simulink model "time_gongji_KVHonline_daoyuan_huace"  (R2019b)
settings: Solver=ode3  StartTime=0.0  StopTime=6000  FixedStep=0.01  MaxStep=0.01  RelTol=1e-3
values from neighbouring files (symbols this model uses):
  bias_gyro_z_gongji = 2e-3    (= 0.002)    [sych_ite_KVHonline_daoyuan_huace.m]
  g = 9.8    [sych_ite_KVHonline_daoyuan_huace.m]
settings Model: Creator=luyishi_E480  LastModifiedBy=xie_z
settings DataIOCC: SaveOutput=off  SignalLogging=off  DSMLogging=off  InspectSignalLogs=on  SaveTime=off  ReturnWorkspaceOutputs=off
settings DebuggingCC: InheritedTsInSrcMsg=none

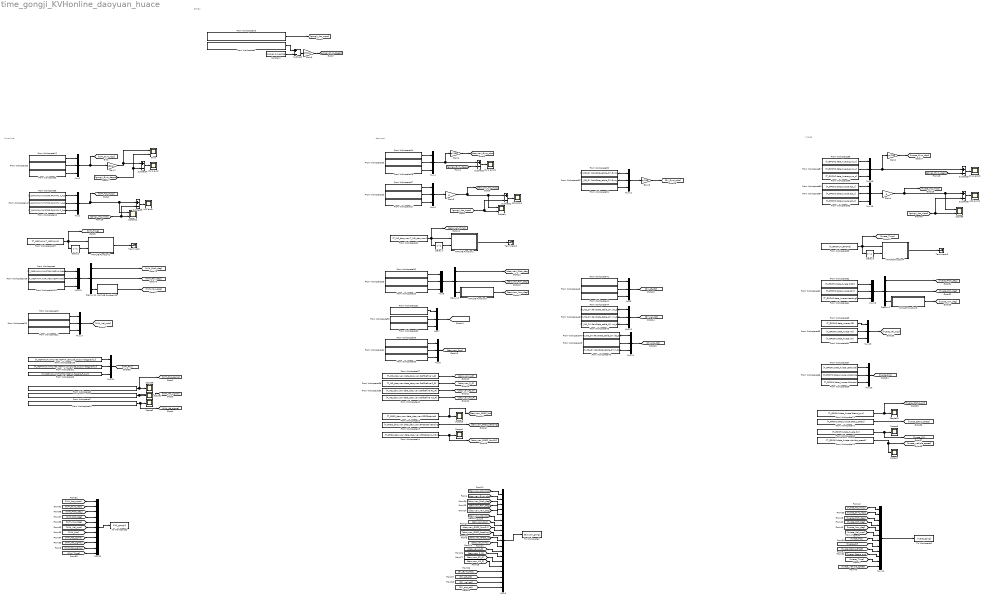
== system time_gongji_KVHonline_daoyuan_huace ==
  note: huace
  note: daoyuan
  note: gongji
  note: kvhonline
  ACC error : Scope
  ACC error1 : Scope
  ACC error2 : Scope
  Constant : Constant  Value=bias_gyro_z_gongji
  Delay1 : Delay  DelayLength=1  InitialCondition=0
  Delay2 : Delay  DelayLength=1  InitialCondition=0
  Delay3 : Delay  DelayLength=1  InitialCondition=0
  Demux1 : Demux  Outputs=3
  Demux14 : Demux  Outputs=3
  Demux2 : Demux  Outputs=3
  From Workspace1 : FromWorkspace  VariableName=[T_INSPVAXA,KVH1750.INSPVA.Longitude_Fusion*deg2rad(1)]  OutputAfterFinalValue=Holding final value
  From Workspace10 : FromWorkspace  VariableName=[T_RAWIMU,KVH1750.RAWIMU.Z_Acc]  Interpolate=off  OutputAfterFinalValue=Holding final value
  From Workspace103 : FromWorkspace  VariableName=[T_INSPVAXA,KVH1750.INSPVA.Latitude_Fusion*deg2rad(1)]  OutputAfterFinalValue=Holding final value
  From Workspace108 : FromWorkspace  VariableName=[T_INSPVAXA,KVH1750.INSPVA.Roll]  Interpolate=off  OutputAfterFinalValue=Holding final value
  From Workspace109 : FromWorkspace  VariableName=[T_INSPVAXA,T_INSPVAXA]  Interpolate=off  OutputAfterFinalValue=Holding final value
  From Workspace11 : FromWorkspace  VariableName=[T_RAWIMU,KVH1750.RAWIMU.Y_Acc]  Interpolate=off  OutputAfterFinalValue=Holding final value
  From Workspace110 : FromWorkspace  VariableName=[T_INSPVAXA,KVH1750.INSPVA.Azimuth]  Interpolate=off  OutputAfterFinalValue=Holding final value
  From Workspace12 : FromWorkspace  VariableName=[T_RAWIMU,KVH1750.RAWIMU.X_Gyro]  Interpolate=off  OutputAfterFinalValue=Holding final value
  From Workspace13 : FromWorkspace  VariableName=[T_INSPVAXA,KVH1750.INSPVA.Pitch_sigma_Fusion,KVH1750.INSPVA.Roll_sigma_Fusion,KVH1750.INSPVA.Azimuth_sigma_Fusion]  Interpolate=off  OutputAfterFinalValue=Holding final value
  From Workspace14 : FromWorkspace  VariableName=[T_GNSS_daoyuan,data_daoyuan.GPSData.NumSV]  Interpolate=off  OutputAfterFinalValue=Holding final value
  From Workspace15 : FromWorkspace  VariableName=[T_GNSS_daoyuan,data_daoyuan.GPSData.heading]  Interpolate=off  OutputAfterFinalValue=Holding final value
  From Workspace16 : FromWorkspace  VariableName=[T_GNSS_daoyuan,data_daoyuan.GPSData.Lat]  Interpolate=off  OutputAfterFinalValue=Holding final value
  From Workspace17 : FromWorkspace  VariableName=[T_INS_daoyuan,-data_daoyuan.INSData.a(:,3)]  Interpolate=off  OutputAfterFinalValue=Holding final value
  From Workspace18 : FromWorkspace  VariableName=[Time,RawData_table.IMU_ACC_x,RawData_table.IMU_ACC_y,RawData_table.IMU_ACC_z]  Interpolate=off  OutputAfterFinalValue=Holding final value
  From Workspace19 : FromWorkspace  VariableName=[T_INSPVAXA,KVH1750.INSPVA.Vel_E_Fusion]  Interpolate=off  OutputAfterFinalValue=Holding final value
  From Workspace2 : FromWorkspace  VariableName=[Time,RawData_table.IMU_Gyro_x,RawData_table.IMU_Gyro_y,RawData_table.IMU_Gyro_z]  Interpolate=off  OutputAfterFinalValue=Holding final value
  From Workspace20 : FromWorkspace  VariableName=[T_INSPVAXA,KVH1750.INSPVA.Vel_N_Fusion]  Interpolate=off  OutputAfterFinalValue=Holding final value
  From Workspace21 : FromWorkspace  VariableName=[T_INSPVAXA,KVH1750.INSPVA.Vel_U_Fusion]  Interpolate=off  OutputAfterFinalValue=Holding final value
  From Workspace22 : FromWorkspace  VariableName=[T_INS_daoyuan,T_INS_daoyuan]  Interpolate=off  OutputAfterFinalValue=Holding final value
  From Workspace23 : FromWorkspace  VariableName=[T_INS_daoyuan,data_daoyuan.INSData.a(:,1)]  Interpolate=off  OutputAfterFinalValue=Holding final value
  From Workspace24 : FromWorkspace  VariableName=[T_INS_daoyuan,data_daoyuan.INSData.g(:,2)]  Interpolate=off  OutputAfterFinalValue=Holding final value
  From Workspace25 : FromWorkspace  VariableName=[T_INS_daoyuan,-data_daoyuan.INSData.g(:,3)]  Interpolate=off  OutputAfterFinalValue=Holding final value
  From Workspace26 : FromWorkspace  VariableName=[T_INS_daoyuan,data_daoyuan.INSData.g(:,1)]  Interpolate=off  OutputAfterFinalValue=Holding final value
  From Workspace27 : FromWorkspace  VariableName=[T_INS_daoyuan,data_daoyuan.INSData.a(:,2)]  Interpolate=off  OutputAfterFinalValue=Holding final value
  From Workspace28 : FromWorkspace  VariableName=[T_INS_daoyuan,data_daoyuan.INSData.angle(:,1)]  Interpolate=off  OutputAfterFinalValue=Holding final value
  From Workspace29 : FromWorkspace  VariableName=[T_INS_daoyuan,data_daoyuan.INSData.angle(:,3)]  Interpolate=off  OutputAfterFinalValue=Holding final value
  From Workspace3 : FromWorkspace  VariableName=[T_RAWIMU,KVH1750.RAWIMU.Z_Gyro]  Interpolate=off  OutputAfterFinalValue=Holding final value
  From Workspace30 : FromWorkspace  VariableName=[T_INS_daoyuan,data_daoyuan.INSData.angle(:,2)]  Interpolate=off  OutputAfterFinalValue=Holding final value
  From Workspace31 : FromWorkspace  VariableName=[T_INS_daoyuan,data_daoyuan.INSData.v(:,2)]  Interpolate=off  OutputAfterFinalValue=Holding final value
  From Workspace32 : FromWorkspace  VariableName=[T_INS_daoyuan,-data_daoyuan.INSData.v(:,3)]  Interpolate=off  OutputAfterFinalValue=Holding final value
  From Workspace33 : FromWorkspace  VariableName=[T_INS_daoyuan,data_daoyuan.INSData.v(:,1)]  Interpolate=off  OutputAfterFinalValue=Holding final value
  From Workspace34 : FromWorkspace  VariableName=[T_INS_daoyuan,data_daoyuan.INSData.pos(:,2)]  Interpolate=off  OutputAfterFinalValue=Holding final value
  From Workspace35 : FromWorkspace  VariableName=[T_INS_daoyuan,data_daoyuan.INSData.pos(:,1)]  Interpolate=off  OutputAfterFinalValue=Holding final value
  From Workspace36 : FromWorkspace  VariableName=[T_INS_daoyuan,data_daoyuan.INSData.pos(:,3)]  Interpolate=off  OutputAfterFinalValue=Holding final value
  From Workspace37 : FromWorkspace  VariableName=[T_INS_daoyuan,data_daoyuan.SelfDefine.V_R]  Interpolate=off  OutputAfterFinalValue=Holding final value
  From Workspace38 : FromWorkspace  VariableName=[T_INS_daoyuan,data_daoyuan.SelfDefine.P_R]  Interpolate=off  OutputAfterFinalValue=Holding final value
  From Workspace39 : FromWorkspace  VariableName=[T_INS_daoyuan,data_daoyuan.SelfDefine.R2_R]  Interpolate=off  OutputAfterFinalValue=Holding final value
  From Workspace4 : FromWorkspace  VariableName=[T_INSPVAXA,KVH1750.INSPVA.Pitch]  Interpolate=off  OutputAfterFinalValue=Holding final value
  From Workspace40 : FromWorkspace  VariableName=[T_INS_daoyuan,data_daoyuan.SelfDefine.H2_R]  Interpolate=off  OutputAfterFinalValue=Holding final value
  From Workspace41 : FromWorkspace  VariableName=[T_INS_DY,RawData_table_DY.pitch_std]  Interpolate=off  OutputAfterFinalValue=Holding final value
  From Workspace42 : FromWorkspace  VariableName=[T_INS_DY,RawData_table_DY.yaw_std]  Interpolate=off  OutputAfterFinalValue=Holding final value
  From Workspace43 : FromWorkspace  VariableName=[T_INS_DY,RawData_table_DY.roll_std]  Interpolate=off  OutputAfterFinalValue=Holding final value
  From Workspace44 : FromWorkspace  VariableName=[T_INS_DY,RawData_table_DY.ve_std]  Interpolate=off  OutputAfterFinalValue=Holding final value
  From Workspace45 : FromWorkspace  VariableName=[T_INS_DY,RawData_table_DY.vd_std]  Interpolate=off  OutputAfterFinalValue=Holding final value
  From Workspace46 : FromWorkspace  VariableName=[T_INS_DY,RawData_table_DY.vn_std]  Interpolate=off  OutputAfterFinalValue=Holding final value
  From Workspace47 : FromWorkspace  VariableName=[T_INS_DY,RawData_table_DY.lat_std]  Interpolate=off  OutputAfterFinalValue=Holding final value
  From Workspace48 : FromWorkspace  VariableName=[T_INS_DY,RawData_table_DY.h_std]  Interpolate=off  OutputAfterFinalValue=Holding final value
  From Workspace49 : FromWorkspace  VariableName=[T_INS_DY,RawData_table_DY.long_std]  Interpolate=off  OutputAfterFinalValue=Holding final value
  From Workspace5 : FromWorkspace  VariableName=[T_INSPVAXA,KVH1750.INSPVA.Height_Fusion]  OutputAfterFinalValue=Holding final value
  From Workspace50 : FromWorkspace  VariableName=[T_INS_DY,RawData_table_DY.Gyro_y]  Interpolate=off  OutputAfterFinalValue=Holding final value
  From Workspace51 : FromWorkspace  VariableName=[T_INS_DY,-RawData_table_DY.Gyro_z]  Interpolate=off  OutputAfterFinalValue=Holding final value
  From Workspace52 : FromWorkspace  VariableName=[T_INS_DY,RawData_table_DY.Gyro_x]  Interpolate=off  OutputAfterFinalValue=Holding final value
  From Workspace53 : FromWorkspace  VariableName=[T_GPCHC,data_huace.acc_z]  Interpolate=off  OutputAfterFinalValue=Holding final value
  From Workspace54 : FromWorkspace  VariableName=[T_GPCHC,data_huace.acc_y]  Interpolate=off  OutputAfterFinalValue=Holding final value
  From Workspace55 : FromWorkspace  VariableName=[T_GPCHC,data_huace.gyro_x]  Interpolate=off  OutputAfterFinalValue=Holding final value
  From Workspace56 : FromWorkspace  VariableName=[T_GPCHC,data_huace.gyro_z]  Interpolate=off  OutputAfterFinalValue=Holding final value
  From Workspace57 : FromWorkspace  VariableName=[T_GPCHC,data_huace.gyro_y]  Interpolate=off  OutputAfterFinalValue=Holding final value
  From Workspace58 : FromWorkspace  VariableName=[T_GPCHC,data_huace.acc_x]  Interpolate=off  OutputAfterFinalValue=Holding final value
  From Workspace59 : FromWorkspace  VariableName=[T_GPCHC,T_GPCHC]  Interpolate=off  OutputAfterFinalValue=Holding final value
  From Workspace6 : FromWorkspace  VariableName=[T_RAWIMU,KVH1750.RAWIMU.Y_Gyro]  Interpolate=off  OutputAfterFinalValue=Holding final value
  From Workspace60 : FromWorkspace  VariableName=[T_GPCHC,data_huace.Roll]  Interpolate=off  OutputAfterFinalValue=Holding final value
  From Workspace61 : FromWorkspace  VariableName=[T_GPCHC,data_huace.Heading]  Interpolate=off  OutputAfterFinalValue=Holding final value
  From Workspace62 : FromWorkspace  VariableName=[T_GPCHC,data_huace.Pitch]  Interpolate=off  OutputAfterFinalValue=Holding final value
  From Workspace63 : FromWorkspace  VariableName=[T_GPCHC,data_huace.VE]  Interpolate=off  OutputAfterFinalValue=Holding final value
  From Workspace64 : FromWorkspace  VariableName=[T_GPCHC,data_huace.VU]  Interpolate=off  OutputAfterFinalValue=Holding final value
  From Workspace65 : FromWorkspace  VariableName=[T_GPCHC,data_huace.VN]  Interpolate=off  OutputAfterFinalValue=Holding final value
  From Workspace66 : FromWorkspace  VariableName=[T_GPCHC,data_huace.Longitude]  Interpolate=off  OutputAfterFinalValue=Holding final value
  From Workspace67 : FromWorkspace  VariableName=[T_GPCHC,data_huace.Lattitude]  Interpolate=off  OutputAfterFinalValue=Holding final value
  From Workspace68 : FromWorkspace  VariableName=[T_GPCHC,data_huace.Altitude]  Interpolate=off  OutputAfterFinalValue=Holding final value
  From Workspace69 : FromWorkspace  VariableName=[T_GPCHC,data_huace.SV]  Interpolate=off  OutputAfterFinalValue=Holding final value
  From Workspace7 : FromWorkspace  VariableName=[T_INSPVAXA,KVH1750.INSPVA.Vel_E_sigma_Fusion,KVH1750.INSPVA.Vel_N_sigma_Fusion,KVH1750.INSPVA.Vel_U_sigma_Fusion]  Interpolate=off  OutputAfterFinalValue=Holding final value
  From Workspace70 : FromWorkspace  VariableName=[T_GPCHC,data_huace.vehicle_speed]  Interpolate=off  OutputAfterFinalValue=Holding final value
  From Workspace71 : FromWorkspace  VariableName=[T_GPCHC,data_huace.Status_GNSS]  Interpolate=off  OutputAfterFinalValue=Holding final value
  From Workspace72 : FromWorkspace  VariableName=[T_GPCHC,data_huace.Status_sys]  Interpolate=off  OutputAfterFinalValue=Holding final value
  From Workspace8 : FromWorkspace  VariableName=[T_INSPVAXA,KVH1750.INSPVA.Lat_sigma_Fusion,KVH1750.INSPVA.Long_sigma_Fusion,KVH1750.INSPVA.Height_sigma_Fusion]  Interpolate=off  OutputAfterFinalValue=Holding final value
  From Workspace9 : FromWorkspace  VariableName=[T_RAWIMU,KVH1750.RAWIMU.X_Acc]  Interpolate=off  OutputAfterFinalValue=Holding final value
  Gain1 : Gain  Gain=pi/180
  Gain2 : Gain  Gain=pi/180
  Gain3 : Gain  Gain=g
  Gain4 : Gain  Gain=g
  Gain6 : Gain  Gain=180/pi
  Gain7 : Gain  Gain=180/pi
  Gain8 : Gain  Gain=pi/180
  "Gyro " : Scope  NumInputPorts=2
  Gyro error : Scope
  Gyro error1 : Scope
  Gyro error2 : Scope
  MATLAB Function1 : MATLAB Function  TreatAsAtomicUnit=on
  MATLAB Function10 : MATLAB Function  TreatAsAtomicUnit=on
  MATLAB Function2 : MATLAB Function  TreatAsAtomicUnit=on
  MATLAB Function3 : MATLAB Function  TreatAsAtomicUnit=on
  MATLAB Function4 : MATLAB Function  TreatAsAtomicUnit=on
  MATLAB Function5 : MATLAB Function  TreatAsAtomicUnit=on
  Mux{1..5,7..13,15..20,24} (19 alike) : Mux  Inputs=3
  Mux14 : Mux  Inputs=12
  Mux21 : Mux  Inputs=11
  Mux6 : Mux  Inputs=19
  Scope{1..2,4..5,7..10} (8 alike) : Scope
  Scope12 : Scope  NumInputPorts=2
  Scope3 : Scope  NumInputPorts=2
  Scope6 : Scope  NumInputPorts=2
  Subtract{,1..6} (7 alike) : Sum  Inputs=+-
  Terminator : Terminator
  Terminator1 : Terminator
  Terminator2 : Terminator
  To Workspace1 : ToWorkspace  VariableName=daoyuan_gongji  SaveFormat=Structure With Time  SampleTime=-1
  To Workspace2 : ToWorkspace  VariableName=huace_gongji  SaveFormat=Structure With Time  SampleTime=-1
  To Workspace3 : ToWorkspace  VariableName=KVH_gongji1  SaveFormat=Structure With Time  SampleTime=-1
  wires:
  Mux2/1 -> [KVH_Gyro_rdps], Gain7/1
  Subtract4/1 -> Gyro error/1
  Subtract5/1 -> ACC error/1
  Gain7/1 -> "Gyro "/1, Subtract4/1  "KVH"
  Mux1/1 -> [KVH_Acc_mpss], Subtract5/1, Scope12/1  "KVH"
  From Workspace9/1 -> Mux1/1
  From Workspace11/1 -> Mux1/2
  From Workspace10/1 -> Mux1/3
  From Workspace3/1 -> Mux2/3
  From Workspace6/1 -> Mux2/2
  From Workspace12/1 -> Mux2/1
  Subtract/1 -> Gain6/1
  Constant/1 -> Subtract/2
  From Workspace2/1 -> Subtract/1  "gongji"
  From Workspace18/1 -> [gongji_Acc_mpss]  "gongji"
  Gain6/1 -> [gongji_Gyro_degps]  "gongji"
  [gongji_Gyro_degps] -> Subtract4/2, "Gyro "/2
  [gongji_Acc_mpss] -> Subtract5/2, Scope12/2
  [gongji_Acc_mpss] -> Subtract2/2, Scope3/2  "gongji"
  From Workspace25/1 -> Mux4/3
  From Workspace23/1 -> Mux3/2
  Mux3/1 -> Gain3/1  "KVH"
  [gongji_Gyro_degps] -> Subtract1/2  "gongji"
  Gain3/1 -> [daoyuan_Acc_mpss], Scope3/1, Subtract2/1  "daoyuan"
  Mux4/1 -> Gain2/1, Subtract1/1  "daoyuan"
  From Workspace17/1 -> Mux3/3
  Gain2/1 -> [daoyuan_Gyro_rdps]
  From Workspace24/1 -> Mux4/1
  From Workspace27/1 -> Mux3/1
  Subtract2/1 -> ACC error1/1
  Delay1/1 -> MATLAB Function1/2(x_k_1)
  MATLAB Function1/1(y) -> Terminator1/1
  From Workspace26/1 -> Mux4/2
  Subtract1/1 -> Gyro error1/1
  From Workspace22/1 -> [daoyuan_Time], Delay1/1, MATLAB Function1/1(x)
  MATLAB Function3/1(Heading_ENU) -> [daoyuan_Yaw_deg]
  Demux1/3 -> MATLAB Function3/1(Heading_North)
  Mux5/1 -> Demux1/1
  Demux1/1 -> [daoyuan_Pitch_deg]
  From Workspace30/1 -> Mux5/1
  Demux1/2 -> [daoyuan_Roll_deg]
  From Workspace29/1 -> Mux5/3
  From Workspace28/1 -> Mux5/2
  [DY_Gyro_rdps] -> Mux6/16
  [daoyuan_H2_R] -> Mux6/15
  [daoyuan_P_R] -> Mux6/13
  [daoyuan_GNSS_lat] -> Mux6/10
  [daoyuan_V_R] -> Mux6/12
  [daoyuan_Yaw_deg] -> Mux6/5
  [daoyuan_Vel_mps] -> Mux6/6
  [daoyuan_Pitch_deg] -> Mux6/3
  [daoyuan_Roll_deg] -> Mux6/4
  [daoyuan_R2_R] -> Mux6/14
  [daoyuan_GNSS_heading] -> Mux6/9
  [DY_vel_std] -> Mux6/18
  [daoyuan_GNSS_NumSV] -> Mux6/8
  [daoyuan_Time] -> Mux6/11
  [daoyuan_Pos] -> Mux6/7
  [daoyuan_Acc_mpss] -> Mux6/1
  [daoyuan_Gyro_rdps] -> Mux6/2
  [DY_att_std] -> Mux6/17
  [DY_pos_std] -> Mux6/19
  Mux6/1 -> To Workspace1/1
  From Workspace33/1 -> Mux7/2
  From Workspace31/1 -> Mux7/1
  Mux7/1 -> [daoyuan_Vel_mps]
  From Workspace32/1 -> Mux7/3
  From Workspace34/1 -> Mux8/2
  From Workspace35/1 -> Mux8/1
  Mux8/1 -> [daoyuan_Pos]
  From Workspace36/1 -> Mux8/3
  From Workspace14/1 -> [daoyuan_GNSS_NumSV], Scope4/1
  From Workspace15/1 -> [daoyuan_GNSS_heading]
  From Workspace16/1 -> Scope5/1, [daoyuan_GNSS_lat]
  From Workspace38/1 -> [daoyuan_P_R]
  From Workspace40/1 -> [daoyuan_H2_R]
  From Workspace39/1 -> [daoyuan_R2_R]
  From Workspace37/1 -> [daoyuan_V_R]
  From Workspace44/1 -> Mux10/1
  From Workspace48/1 -> Mux11/3
  From Workspace45/1 -> Mux10/3
  Mux11/1 -> [DY_pos_std]  "DY"
  Mux10/1 -> [DY_vel_std]  "DY"
  From Workspace49/1 -> Mux11/2
  From Workspace47/1 -> Mux11/1
  From Workspace42/1 -> Mux9/3
  From Workspace46/1 -> Mux10/2
  From Workspace41/1 -> Mux9/1
  Mux9/1 -> [DY_att_std]  "DY"
  From Workspace43/1 -> Mux9/2
  From Workspace51/1 -> Mux12/3
  From Workspace52/1 -> Mux12/2
  Mux12/1 -> Gain8/1  "DY"
  Gain8/1 -> [DY_Gyro_rdps]
  From Workspace50/1 -> Mux12/1
  [huace_Acc_mpss] -> Mux14/1
  [huace_SV] -> Mux14/8
  [huace_Time] -> Mux14/11
  [huace_Yaw_deg] -> Mux14/5
  [huace_vehicle_speed] -> Mux14/12
  Mux14/1 -> To Workspace2/1
  [huace_Roll_deg] -> Mux14/4
  [huace_Pitch_deg] -> Mux14/3
  [huace_Pos] -> Mux14/7
  [huace_Status_GNSS] -> Mux14/9
  [huace_Vel_mps] -> Mux14/6
  [huace_Gyro_rdps] -> Mux14/2
  [huace_Status_sys] -> Mux14/10
  From Workspace57/1 -> Mux16/2
  From Workspace53/1 -> Mux15/3
  Subtract6/1 -> ACC error2/1
  [gongji_Gyro_degps] -> Subtract3/2  "gongji"
  Gain4/1 -> [huace_Acc_mpss], Scope6/1, Subtract6/1  "huace"
  Gain1/1 -> [huace_Gyro_rdps]
  From Workspace55/1 -> Mux16/1
  From Workspace54/1 -> Mux15/2
  From Workspace56/1 -> Mux16/3
  From Workspace58/1 -> Mux15/1
  [gongji_Acc_mpss] -> Subtract6/2, Scope6/2  "gongji"
  Mux15/1 -> Gain4/1  "KVH"
  Mux16/1 -> Subtract3/1, Gain1/1  "huace"
  Subtract3/1 -> Gyro error2/1
  MATLAB Function4/1(y) -> Terminator2/1
  From Workspace59/1 -> [huace_Time], Delay3/1, MATLAB Function4/1(x)
  Delay3/1 -> MATLAB Function4/2(x_k_1)
  From Workspace60/1 -> Mux18/2
  From Workspace62/1 -> Mux18/1
  MATLAB Function5/1(Heading_ENU) -> [huace_Yaw_deg]
  Demux2/1 -> [huace_Pitch_deg]
  Demux2/2 -> [huace_Roll_deg]
  Mux18/1 -> Demux2/1
  Demux2/3 -> MATLAB Function5/1(Heading_North)
  From Workspace61/1 -> Mux18/3
  From Workspace63/1 -> Mux19/1
  From Workspace64/1 -> Mux19/3
  From Workspace65/1 -> Mux19/2
  Mux19/1 -> [huace_Vel_mps]
  Mux20/1 -> [huace_Pos]
  From Workspace68/1 -> Mux20/3
  From Workspace66/1 -> Mux20/2
  From Workspace67/1 -> Mux20/1
  From Workspace70/1 -> Scope7/1, [huace_vehicle_speed]
  From Workspace71/1 -> [huace_Status_GNSS]
  From Workspace69/1 -> [huace_SV], Scope9/1
  From Workspace72/1 -> Scope10/1, [huace_Status_sys]
  MATLAB Function2/1(y) -> Terminator/1
  Delay2/1 -> MATLAB Function2/2(x_k_1)
  From Workspace109/1 -> [KVH_Time], Delay2/1, MATLAB Function2/1(x)
  Demux14/1 -> [KVH_Pitch_deg]
  From Workspace4/1 -> Mux13/1
  Demux14/3 -> MATLAB Function10/1(Heading_North)
  Demux14/2 -> [KVH_Roll_deg]
  From Workspace110/1 -> Mux13/3
  From Workspace108/1 -> Mux13/2
  Mux13/1 -> Demux14/1
  MATLAB Function10/1(Heading_ENU) -> [KVH_Yaw_deg]
  From Workspace21/1 -> Mux17/3
  From Workspace19/1 -> Mux17/1
  From Workspace20/1 -> Mux17/2
  Mux17/1 -> [KVH_Vel_mps]
  From Workspace5/1 -> Mux24/3
  From Workspace7/1 -> [KVH_Vel_sigma], Scope1/1
  From Workspace13/1 -> [KVH_Att_sigma], Scope2/1
  Mux24/1 -> [KVH_Pos]
  From Workspace103/1 -> Mux24/1
  From Workspace1/1 -> Mux24/2
  From Workspace8/1 -> [KVH_Pos_sigma], Scope8/1
  [KVH_Pos_sigma] -> Mux21/10
  [KVH_Att_sigma] -> Mux21/8
  [KVH_Acc_mpss] -> Mux21/1
  Mux21/1 -> To Workspace3/1
  [KVH_Pitch_deg] -> Mux21/3
  [KVH_Time] -> Mux21/11
  [KVH_Vel_mps] -> Mux21/6
  [KVH_Yaw_deg] -> Mux21/5
  [KVH_Roll_deg] -> Mux21/4
  [KVH_Pos] -> Mux21/7
  [KVH_Gyro_rdps] -> Mux21/2
  [KVH_Vel_sigma] -> Mux21/9

== matlab function time_gongji_KVHonline_daoyuan_huace/MATLAB Function1 ==
  data: y output; x input; x_k_1 input
function y  = fcn(x,x_k_1)
    if x ~= x_k_1
        y = uint8(1);
    else
        y = uint8(0);
    end
end

== matlab function time_gongji_KVHonline_daoyuan_huace/MATLAB Function3 ==
  data: Heading_North input; Heading_ENU output size=1
function Heading_ENU = fcn(Heading_North)
% Heading_ENU:以北为零顺时针为正0-360°
% Heading_North:以北为零逆时针为正-180-180°

% Heading_North = Heading_North + 0.5 + 3.8;
if Heading_North <= 180
    Heading_ENU = 0 - Heading_North;
else
    Heading_ENU = 360 - Heading_North;
end

== matlab function time_gongji_KVHonline_daoyuan_huace/MATLAB Function4 ==
  data: y output; x input; x_k_1 input
function y  = fcn(x,x_k_1)
    if x ~= x_k_1
        y = uint8(1);
    else
        y = uint8(0);
    end
end

== matlab function time_gongji_KVHonline_daoyuan_huace/MATLAB Function5 ==
  data: Heading_North input; Heading_ENU output size=1
function Heading_ENU = fcn(Heading_North)
% Heading_ENU:以北为零顺时针为正0-360°
% Heading_North:以北为零逆时针为正-180-180°

% Heading_North = Heading_North + 0.5 + 3.8;
if Heading_North <= 180
    Heading_ENU = 0 - Heading_North;
else
    Heading_ENU = 360 - Heading_North;
end

== matlab function time_gongji_KVHonline_daoyuan_huace/MATLAB Function2 ==
  data: y output; x input; x_k_1 input
function y  = fcn(x,x_k_1)
    if x ~= x_k_1
        y = uint8(1);
    else
        y = uint8(0);
    end
end

== matlab function time_gongji_KVHonline_daoyuan_huace/MATLAB Function10 ==
  data: Heading_North input; Heading_ENU output size=1
function Heading_ENU = fcn(Heading_North)
% Heading_ENU:以北为零顺时针为正0-360°
% Heading_North:以北为零逆时针为正-180-180°

% Heading_North = Heading_North + 0.5 + 3.8;
if Heading_North <= 180
    Heading_ENU = 0 - Heading_North;
else
    Heading_ENU = 360 - Heading_North;
end
